simulink model "do_alef_be"  (R2020a)
settings: Solver=VariableStepAuto  StartTime=0.0  StopTime=25  FixedStep=0.01
settings Model: Creator=ASUS  LastModifiedBy=Javad
settings DebuggingCC: UnconnectedInputMsg=none  UnconnectedOutputMsg=none  UnconnectedLineMsg=none
settings ModelReferenceCC: EnableRefExpFcnMdlSchedulingChecks=off
settings RTWCC: Description=Generic Real-Time Target

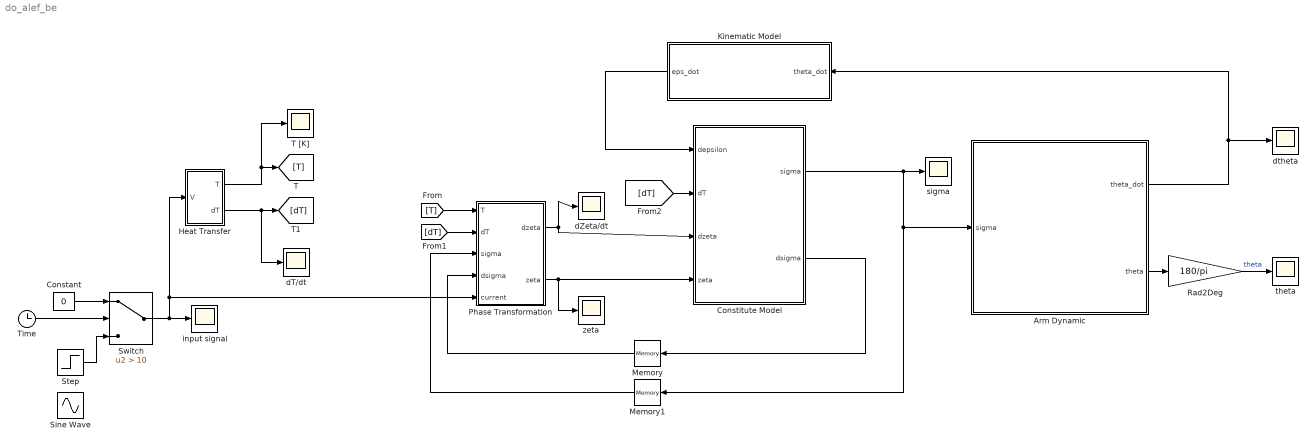
== system do_alef_be ==
  Arm Dynamic : Subsystem
  Constant : Constant  Value=0
  Constitute Model : Subsystem
  Heat Transfer : Subsystem
  Kinematic Model : MATLAB Function  TreatAsAtomicUnit=on
  Memory : Memory
  Memory1 : Memory  InitialCondition=75e6
  Phase Transformation : Subsystem
  Rad2Deg : Gain  Gain=180/pi
  Sine Wave : Sin  Amplitude=25  Frequency=2*pi/10  SampleTime=0
  Step : Step  After=20  SampleTime=0
  Switch : Switch  Criteria=u2 > Threshold  Threshold=10
  T [K] : Scope
  Time : Clock
  dT/dt : Scope
  dZeta/dt : Scope
  dtheta : Scope
  input signal : Scope
  sigma : Scope
  theta : Scope
  zeta : Scope
  wires:
  Arm Dynamic/2(theta) -> Rad2Deg/1
  Arm Dynamic/1(theta_dot) -> Kinematic Model/1(theta_dot), dtheta/1
  Phase Transformation/1(dzeta) -> dZeta/dt/1, Constitute Model/3(dzeta)
  [T] -> Phase Transformation/1(T)
  [dT] -> Phase Transformation/2(dT)
  [dT] -> Constitute Model/2(dT)
  Kinematic Model/1(eps_dot) -> Constitute Model/1(depsilon)
  Constitute Model/1(sigma) -> Arm Dynamic/1(sigma), Memory1/1, sigma/1
  Constitute Model/2(dsigma) -> Memory/1
  Rad2Deg/1 -> theta/1  "theta"
  Heat Transfer/1(T) -> T [K]/1, [T]
  Heat Transfer/2(dT) -> dT/dt/1, [dT]
  Phase Transformation/2(zeta) -> zeta/1, Constitute Model/4(zeta)
  Memory1/1 -> Phase Transformation/3(sigma)
  Memory/1 -> Phase Transformation/4(dsigma)
  Time/1 -> Switch/2
  Switch/1 -> input signal/1, Heat Transfer/1(V), Phase Transformation/5(current)
  Constant/1 -> Switch/1
  Step/1 -> Switch/3

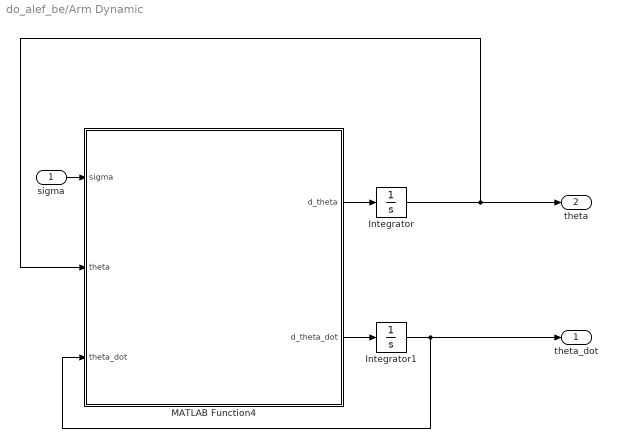
== system do_alef_be/Arm Dynamic ==
  sigma : Inport
  Integrator : Integrator
  Integrator1 : Integrator
  MATLAB Function4 : MATLAB Function  TreatAsAtomicUnit=on
  theta_dot : Outport
  theta : Outport  Port=2
  wires:
  sigma/1 -> MATLAB Function4/1(sigma)
  MATLAB Function4/2(d_theta_dot) -> Integrator1/1
  Integrator/1 -> theta/1, MATLAB Function4/2(theta)
  MATLAB Function4/1(d_theta) -> Integrator/1
  Integrator1/1 -> theta_dot/1, MATLAB Function4/3(theta_dot)

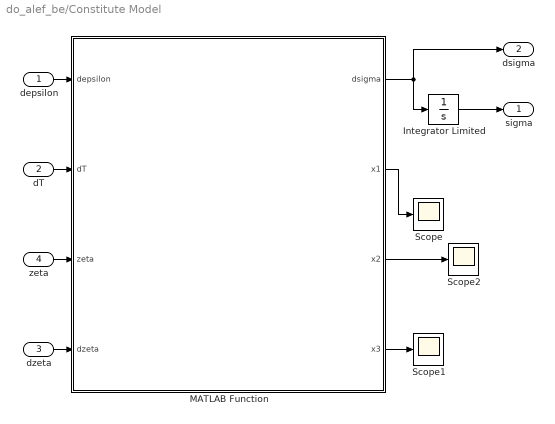
== system do_alef_be/Constitute Model ==
  depsilon : Inport
  dT : Inport  Port=2
  dzeta : Inport  Port=3
  zeta : Inport  Port=4
  Integrator Limited : Integrator  InitialCondition=75*1e6  LimitOutput=on  UpperSaturationLimit=100*1e8  LowerSaturationLimit=0
  MATLAB Function : MATLAB Function  TreatAsAtomicUnit=on
  Scope : Scope
  Scope1 : Scope
  Scope2 : Scope
  sigma : Outport
  dsigma : Outport  Port=2
  wires:
  dzeta/1 -> MATLAB Function/4(dzeta)
  MATLAB Function/1(dsigma) -> dsigma/1, Integrator Limited/1
  zeta/1 -> MATLAB Function/3(zeta)
  depsilon/1 -> MATLAB Function/1(depsilon)
  dT/1 -> MATLAB Function/2(dT)
  Integrator Limited/1 -> sigma/1
  MATLAB Function/3(x2) -> Scope2/1
  MATLAB Function/4(x3) -> Scope1/1
  MATLAB Function/2(x1) -> Scope/1

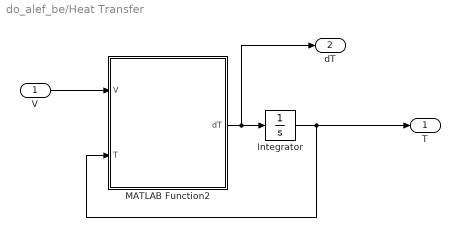
== system do_alef_be/Heat Transfer ==
  V : Inport
  Integrator : Integrator  InitialCondition=298.1500
  MATLAB Function2 : MATLAB Function  TreatAsAtomicUnit=on
  T : Outport
  dT : Outport  Port=2
  wires:
  Integrator/1 -> T/1, MATLAB Function2/2(T)
  MATLAB Function2/1(dT) -> dT/1, Integrator/1
  V/1 -> MATLAB Function2/1(V)

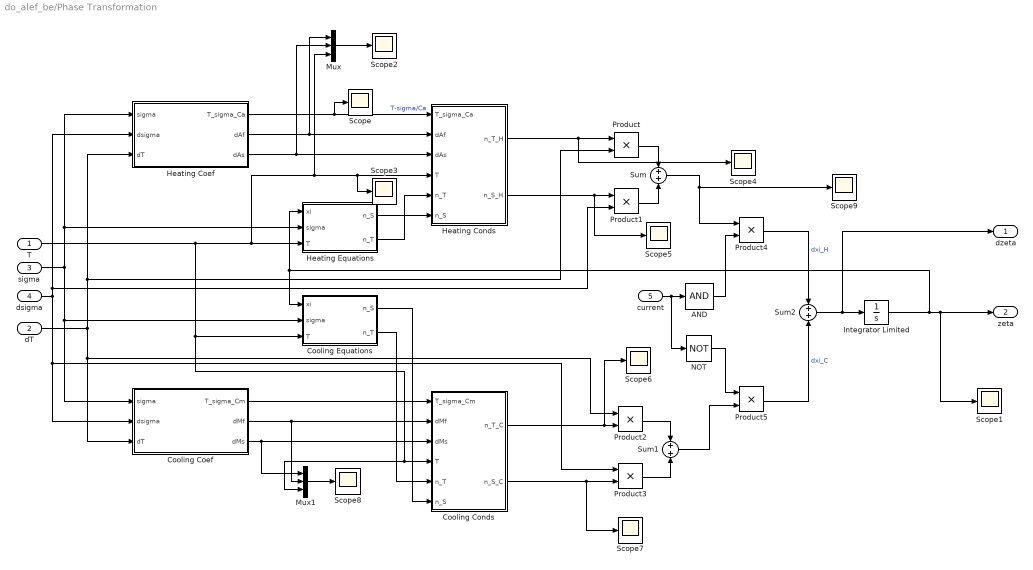
== system do_alef_be/Phase Transformation ==
  T : Inport
  dT : Inport  Port=2
  sigma : Inport  Port=3
  dsigma : Inport  Port=4
  current : Inport  Port=5
  AND : Logic  Inputs=1  IconShape=distinctive  AllPortsSameDT=off  OutDataTypeStr=boolean
  Cooling Coef : MATLAB Function  TreatAsAtomicUnit=on
  Cooling Conds : MATLAB Function  TreatAsAtomicUnit=on
  Cooling Equations : MATLAB Function  TreatAsAtomicUnit=on
  Heating Coef : MATLAB Function  TreatAsAtomicUnit=on
  Heating Conds : MATLAB Function  TreatAsAtomicUnit=on
  Heating Equations : MATLAB Function  TreatAsAtomicUnit=on
  Integrator Limited : Integrator  InitialCondition=0.02  LimitOutput=on  UpperSaturationLimit=1  LowerSaturationLimit=0
  Mux : Mux  Inputs=3
  Mux1 : Mux  Inputs=3
  NOT : Logic  Operator=NOT  IconShape=distinctive  AllPortsSameDT=off  OutDataTypeStr=boolean
  Product{,1..5} (6 alike) : Product
  Scope{,1..9} (10 alike) : Scope
  Sum : Sum  Inputs=+|+
  Sum1 : Sum  Inputs=+|+
  Sum2 : Sum  Inputs=+|+
  dzeta : Outport
  zeta : Outport  Port=2
  wires:
  dT/1 -> Product/2, Heating Coef/3(dT), Product2/1, Cooling Coef/3(dT)
  sigma/1 -> Heating Equations/2(sigma), Heating Coef/1(sigma), Cooling Equations/2(sigma), Cooling Coef/1(sigma)
  dsigma/1 -> Product1/2, Heating Coef/2(dsigma), Product3/1, Cooling Coef/2(dsigma)
  T/1 -> Mux/3, Scope3/1, Heating Conds/4(T), Heating Equations/3(T), Mux1/3, Cooling Conds/4(T), Cooling Equations/3(T)
  Heating Equations/1(n_S) -> Heating Conds/6(n_S)
  Heating Equations/2(n_T) -> Heating Conds/5(n_T)
  Heating Coef/3(dAs) -> Mux/2, Heating Conds/3(dAs)
  Heating Coef/2(dAf) -> Heating Conds/2(dAf), Mux/1
  Heating Coef/1(T_sigma_Ca) -> Scope/1, Heating Conds/1(T_sigma_Ca)  "T-sigma/Ca"
  Cooling Coef/1(T_sigma_Cm) -> Cooling Conds/1(T_sigma_Cm)
  Cooling Equations/1(n_S) -> Cooling Conds/6(n_S)
  Cooling Equations/2(n_T) -> Cooling Conds/5(n_T)
  Cooling Coef/2(dMf) -> Mux1/2, Cooling Conds/2(dMf)
  Cooling Coef/3(dMs) -> Mux1/1, Cooling Conds/3(dMs)
  Heating Conds/1(n_T_H) -> Scope4/1, Product/1
  Heating Conds/2(n_S_H) -> Scope5/1, Product1/1
  Product1/1 -> Sum/2
  Product/1 -> Sum/1
  Cooling Conds/1(n_T_C) -> Scope6/1, Product2/2
  Cooling Conds/2(n_S_C) -> Scope7/1, Product3/2
  Product3/1 -> Sum1/2
  Product2/1 -> Sum1/1
  current/1 -> NOT/1, AND/1
  AND/1 -> Product4/2
  Sum/1 -> Product4/1, Scope9/1
  Sum1/1 -> Product5/2
  NOT/1 -> Product5/1
  Product5/1 -> Sum2/2  "dxi_C"
  Product4/1 -> Sum2/1  "dxi_H"
  Sum2/1 -> dzeta/1, Integrator Limited/1
  Integrator Limited/1 -> Heating Equations/1(xi), Cooling Equations/1(xi), Scope1/1, zeta/1
  Mux/1 -> Scope2/1
  Mux1/1 -> Scope8/1

== matlab function do_alef_be/Phase Transformation/Heating Conds ==
  data: T_sigma_Ca input; n_T_H output; dAf input; dAs input; T input; n_T input; n_S input; n_S_H output
function [n_T_H, n_S_H] = heatingConds(T_sigma_Ca, dAf, dAs, T, n_T, n_S)

if T_sigma_Ca>0 && dAs<=T && T<=dAf
    n_T_H = n_T;
    n_S_H = n_S;
else
    n_T_H = 0;
    n_S_H = 0;
end

end

== matlab function do_alef_be/Phase Transformation/Cooling Conds ==
  data: T_sigma_Cm input; n_T_C output; dMf input; dMs input; T input; n_T input; n_S input; n_S_C output
function [n_T_C, n_S_C] = coolingConds(T_sigma_Cm, dMf, dMs, T, n_T, n_S)

if T_sigma_Cm<0 && dMf<=T && T<=dMs
    n_T_C = n_T;
    n_S_C = n_S;
else
    n_T_C = 0;
    n_S_C = 0;
end

end

== matlab function do_alef_be/Kinematic Model ==
  data: theta_dot input; eps_dot output
function eps_dot = KinematicModel(theta_dot)
%#codegen
% Kinematic model: convert joint angular velocity to SMA strain rate
%
% Inputs:
%   theta_dot  - joint angular velocity (rad/s)
%
% Outputs:
%   eps_dot    - SMA strain rate (1/s)

    % --- ثابت‌های داخلی بلوک (پارامترها) ---
    rp = 8.25e-3;    % شعاع قرقره (m) – مقدار نمونه، بر حسب داده‌های شما
    l0 = 0.9; % طول اولیه سیم SMA (m)
    
    % --- محاسبه نرخ کرنش ---
    eps_dot = -2 * rp / l0 * theta_dot;
end

== matlab function do_alef_be/Constitute Model/MATLAB Function ==
  data: depsilon input; dT input; dsigma output; zeta input; dzeta input; x1 output; x2 output; x3 output
function [dsigma,x1,x2,x3] = SMAConstitutiveModel(depsilon, dT, zeta, dzeta)
% SMAConstitutiveModel   Compute stress‐rate for a one‐variable SMA
%
%   Inputs:
%     depsilon = dε/dt          [1/s]
%     dT       = dT/dt          [K/s]
%     zeta     = ξ              (martensite fraction, dimensionless)
%     dzeta    = dξ/dt          [1/s]
%
%   Outputs:
%     dsigma   = dσ/dt          [Pa/s]
%     zeta_out = ξ (just echoes current zeta for monitoring)
%
%   Constitutive Eq. (Eq. 3):
%     σ̇ = D(ζ)·ε̇  +  θ_T·Ṫ  +  Δ·ζ̇
%     where
%       D(ζ) = ζ·D_A + (1 − ζ)·D_M,
%       Δ    = − D(ζ) · ε₀,
%       θ_T  = thermal‐expansion coefficient (Pa/K).
%
%   NOTE: We assume ε₀ > 0 is the maximum transformation strain.

 %#ok<*NASGU>
 
 % Young’s moduli in Pa (the original had MPa; convert: ×10^6):
 D_A = 75e9;     % 75 GPa (austenite)
 D_M = 38e9;     % 38 GPa (martensite)
 
 % Thermal expansion coefficient (Pa/K):
 theta_T   = 0.55*1e6;   % 0.55 MPa/°C → 0.55×10^6 Pa/K
 
 % Maximum transformation strain ε₀ (dimensionless):
 epsilon_0 = 0.04;      % 4% (typical for NiTi wire)
 
 %--- MIXED MODULUS AND Δ COUPLING TERM ---
 D_mixed = zeta * D_A + (1 - zeta) * D_M;
 Delta   = - D_mixed * epsilon_0;  % Δ = −D·ε₀
 
 %--- STRESS RATE (Eq. 3) ---
 dsigma = (D_mixed * depsilon + theta_T * dT + Delta * dzeta)*1.0;
 
 %--- PASS zeta THROUGH FOR MONITORING ---
 x1 =D_mixed * depsilon;
 x2 = theta_T * dT;
 x3 = Delta * dzeta;
end

== matlab function do_alef_be/Heat Transfer/MATLAB Function2 ==
  data: V input; dT output; T input
function dT  = SMAHeatTransfer(V, T)
%#codegen
% SMA wire heat transfer model based on provided parameters
% Inputs:
%   I - current (Amps)
% Outputs:
%   T - temperature (K)
%   dT_dt - temperature rate (K/s)


% Parameters:
rho = 6.454*1e3;
l_0 = 0.9;
A = pi * (0.3*1e-3)^2/4;
m = rho * A;
% m_gram = 0.0872;           % جرم کل سیم (گرم)
% m = m_gram / 1000;         % جرم به کیلوگرم

cp_kcal = 0.2;            % گرمای ویژه (kcal/kg-C)
cp = cp_kcal * 4184;       % تبدیل به J/kg-K

R_per_length = 48;         % مقاومت سیم (Ohm) (مقاومت کل برای طول سیم)

R = R_per_length;          % مقاومت کل سیم (تقریباً مقاومت داده شده است)
% توجه: در صورت نیاز می‌توان به R = R_per_length * l تغییر داد

Ac_cm2 = 4.345;              % مساحت محیطی سیم (سانتی‌متر مربع)
Ac = Ac_cm2 * 1e-4;        % تبدیل به متر مربع

T_inf_C = 25;              % دمای محیط (سانتی‌گراد)
T_inf = T_inf_C + 273.15;  % تبدیل به کلوین

h0 = 150;                  % ضریب انتقال حرارت پایه (W/m^2-K)
h2 = 0;                    % ضریب درجه دوم ضریب انتقال حرارت (پیشفرض صفر)

% محاسبه ضریب انتقال حرارت با فرض مدل درجه دوم
h = h0 + h2 * T^2;

% محاسبه نرخ تغییر دما بر اساس معادله حرارتی
% m در اینجا جرم کل در نظر گرفته شده است (نه بر واحد طول)
dT = ( (V^2) / R - h * Ac * (T - T_inf) ) / (m * cp);



end

== matlab function do_alef_be/Arm Dynamic/MATLAB Function4 ==
  data: d_theta output; d_theta_dot output; sigma input; theta input; theta_dot input
function [d_theta, d_theta_dot] = ArmDynamicsFromStress(sigma, theta, theta_dot)
%#codegen
% Arm dynamics driven by wire stress σ

% --- پارامترهای داخلی بلوک (از جدول) ---
% قطر سیم 150 µm → سطح مقطع
A_wire = pi*(0.3*1e-3)^2/4;      % (m^2)
% قرقره
rp    = 8.25e-3;                  % قطر قرقره (m)

% گشتاور سیم = σ * A_wire * rp
tau_w_factor = A_wire * rp;    % پیش‌ضرب σ

% وزن بازو+گریپر → گشتاور گرانشی
m_arm = 0.0872;                   % جرم معادل بازو+گریپر (kg) – مثال
m_load = 0.0287;
Lc    = 0.4;                   % مرکز جرم تا مفصل (m) – مثال
g     = 9.81;                  % شتاب گرانش (m/s^2)


% فنر بایاس
k_bias = 0.03015;              % سختی فنر بایاس (N·m/rad)

% میرایی و اینرسی
% I_e    = 0.0872e-3 * (0.3e-3)^2; % تقریب ممان اینرسی سیم + بازو (kg·m^2)
c_damp = 1;                  % ضریب میرایی (N·m·s/rad) – مثال


% --- محاسبه گشتاورها ---
tau_w = sigma * tau_w_factor;               % SMA torque
tau_g = (m_arm * Lc / 2 + m_load * Lc) * g * sin(theta); % gravitational torque
l_spring_initial = 0.04;
l_spring_current = sqrt(2*(Lc/2)^2-2*(Lc/2)^2*cos(theta))+l_spring_initial;
tau_s = k_bias * (l_spring_current-l_spring_initial);       % bias spring torque

I = m_load * Lc^2 + m_arm * (Lc / 2)^2;
% --- معادله دینامیک بازو ---
d_theta_dot = (tau_w - tau_g - tau_s - c_damp * theta_dot) / I;
d_theta     = theta_dot;

end

== matlab function do_alef_be/Phase Transformation/Heating Coef ==
  data: sigma input; dsigma input; dT input; T_sigma_Ca output; dAf output; dAs output
function [T_sigma_Ca, dAf, dAs] = heating_coef(sigma, dsigma, dT)
CA = 10.3e6; 

As = 69  + 273.15;   % 79 °C → 352.15 K
Af = 79  + 273.15;   % 55 °C → 328.15 K

T_sigma_Ca = dT - 1/CA * dsigma;
dAf = sigma / CA + Af;
dAs = sigma / CA + As;
end

== matlab function do_alef_be/Phase Transformation/Cooling Coef ==
  data: sigma input; dsigma input; dT input; T_sigma_Cm output; dMf output; dMs output
function [T_sigma_Cm, dMf, dMs] = cooling_coef(sigma,dsigma, dT)
CM = 10.3e6;

Ms = 55  + 273.15;   % 45 °C → 318.15 K
Mf = 45  + 273.15;   % 69 °C → 342.15 K

T_sigma_Cm = -dT + 1/CM * dsigma;
dMf = sigma / CM + Mf;
dMs = sigma / CM + Ms;

end

== matlab function do_alef_be/Phase Transformation/Heating Equations ==
  data: xi input; n_S output; sigma input; T input; n_T output
function [n_S, n_T] = heatingEq(xi, sigma, T)
CA = 10.3e6; 

As = 79  + 273.15;   % 79 °C → 352.15 K
Af = 55  + 273.15;   % 55 °C → 328.15 K


aA = pi / (Af - As);

arg = (T - (sigma / CA + As))  * aA;

n_T = -0.5 * xi * sin(arg) * aA;

n_S = 0.5 * xi * sin(arg) * aA / CA;

end

== matlab function do_alef_be/Phase Transformation/Cooling Equations ==
  data: xi input; n_S output; sigma input; T input; n_T output
function [n_S, n_T] = coolingEq(xi, sigma, T)
Ms = 45  + 273.15;   % 45 °C → 318.15 K
Mf = 69  + 273.15;   % 69 °C → 342.15 K

CM = 10.3e6;        

aM = pi / (Ms - Mf);

arg = (T - (sigma / CM + Mf))  * aM;

n_T = -0.5 * (1-xi) * sin(arg) * aM;

n_S = 0.5 * (1-xi) * sin(arg) * aM / CM;

end
